simulink model "xindiandao030403"  (R2019a)
settings: Solver=VariableStepAuto  StartTime=0.0  StopTime=30  RelTol=1e-3
libraries: commrandsrc3 x1
settings Model: Creator=Zezzid  LastModifiedBy=Zezzid

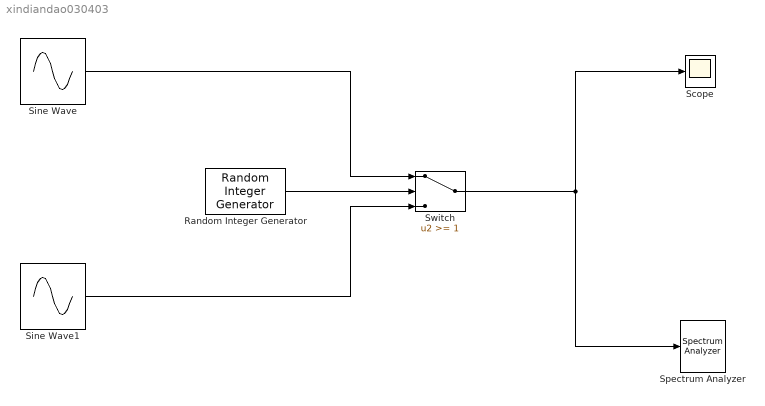
== system xindiandao030403 ==
  Random Integer Generator : commrandsrc3/Random Integer Generator  SetSize=2  SeedSource=Auto  Seed=0  SampleTime=1  SamplesPerFrame=1  OutputDataType=single  SimulateUsing=Code generation
      settings: SourceProductName=Communications Toolbox
  Scope : Scope
  Sine Wave : Sin  Frequency=2*pi*10  SampleTime=1/100
  Sine Wave1 : Sin  Frequency=2*pi*5  SampleTime=1/100
  Spectrum Analyzer : SpectrumAnalyzer
  Switch : Switch  Threshold=1
  wires:
  Sine Wave/1 -> Switch/1
  Random Integer Generator/1 -> Switch/2
  Switch/1 -> Spectrum Analyzer/1, Scope/1
  Sine Wave1/1 -> Switch/3
